simulink model "modelo"  (Simulink 9.1)
settings: Solver=ode15s  StartTime=0.0  StopTime=inf  RelTol=1e-6  EnableMultiTasking=on
libraries: dsparch4 x12, dspmathops x11, dspobslib x7, dspvision x2, dspindex x1
settings Model: Creator=USUARIO  LastModifiedBy=valen
settings DataIOCC: LimitDataPoints=on  SignalLoggingSaveFormat=ModelDataLogs  SignalLoggingName=sigsOut
settings OptimizationCC: ExpressionDepthLimit=2147483647  InitFltsAndDblsToZero=on
settings DebuggingCC: SaveWithParameterizedLinksMsg=none  SignalResolutionControl=TryResolveAllWithWarning  MultiTaskDSMMsg=warning  MultiTaskCondExecSysMsg=none  FcnCallInpInsideContextMsg=warning  StateNameClashWarn=warning
settings HardwareCC: TargetUnknown=on
settings GRTTargetCC: TargetFcnLib=ansi_tfl_tmw.mat

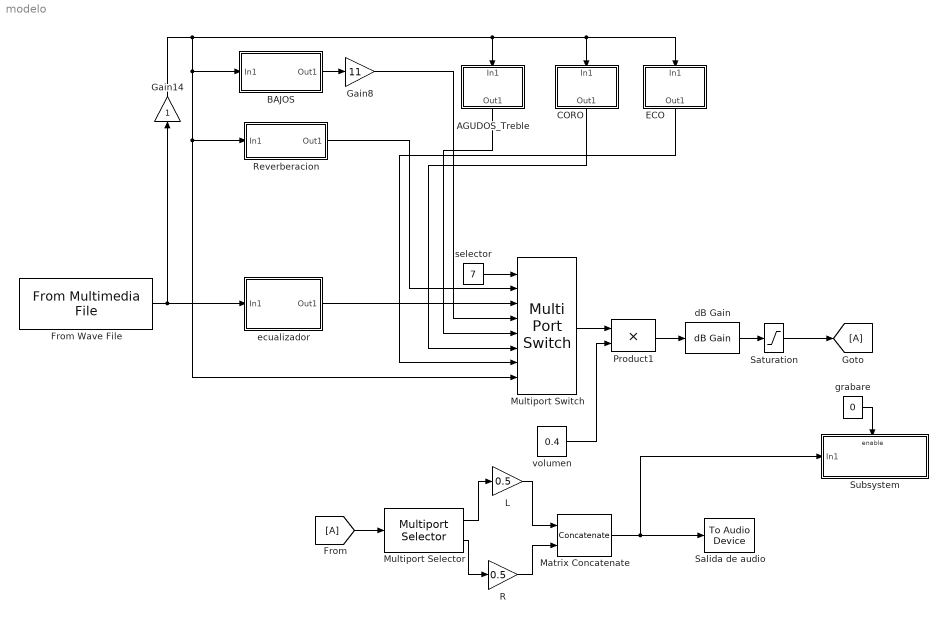
== system modelo ==
  AGUDOS_Treble : Subsystem
  BAJOS : Subsystem
  CORO : Subsystem
  ECO : Subsystem
  From Wave File : dspvision/From Multimedia File  inputFilename=X:\prueba\UNR Ing electrónica\Materias\5.Sistemas y señales I\Unidades\Creo que amo matlab\Ecualizador\5.Ecualizador\LGANTE.wav  loop=on  numPlays=1  outputStreams=Audio only  videoDataType=single  audioDataType=double  inheritSampleTime=on  userDefinedSampleTime=1/30  noAudioOutput=off  isIntensityVideo=off  fourcc=RGB  colorVideoFormat=Separate color signals  outputEOF=off  dataOrg=Column-major  audioFrameSize=256  computeAudioFrameSize=off  outSamplingMode=Frame based
      settings: SourceProductBaseCode=VP
  Gain14 : Gain  SaturateOnIntegerOverflow=on  OutDataTypeStr=Inherit: Same as input  ParamDataTypeStr=Inherit: Same as input
  Gain8 : Gain  Gain=11  SaturateOnIntegerOverflow=on  OutDataTypeStr=Inherit: Same as input  ParamDataTypeStr=Inherit: Same as input
  L : Gain  Gain=0.5
  Matrix Concatenate : Concatenate  Mode=Multidimensional array  ConcatenateDimension=2
  Multiport Selector : dspindex/Multiport Selector  rowsOrCols=Columns  idxCellArray={1,2}  idxErrMode=Clip and Warn
  Multiport Switch : MultiPortSwitch  Inputs=7  SaturateOnIntegerOverflow=on
  Product1 : Product  SaturateOnIntegerOverflow=on  OutDataTypeStr=Inherit: Same as first input
  R : Gain  Gain=0.5
  Reverberacion : Subsystem
  Salida de audio : dspobslib/To Audio Device  deviceName=Default  inheritSampleRate=on  sampleRate=44100  deviceDatatype=Determine from input data type  autoBufferSize=on  bufferSize=4096  queueDuration=2  defaultOutputChannelMapping=on  outputChannelMapping=1:2  outputNumUnderrunSamples=off
      settings: SourceProductName=DSP System Toolbox  SourceProductBaseCode=DS
  Saturation : Saturate  UpperLimit=5  LowerLimit=-5  LinearizeAsGain=off  ZeroCross=off
  Subsystem : Subsystem
  dB Gain : dspmathops/dB Gain  dB=5  intype=Amplitude
      settings: SourceProductName=DSP System Toolbox  SourceProductBaseCode=DS
  ecualizador : Subsystem
  grabare : Constant  Value=0
  selector : Constant  Value=7
  volumen : Constant  Value=0.4
  wires:
  selector/1 -> Multiport Switch/1
  Multiport Switch/1 -> Product1/1
  Product1/1 -> dB Gain/1
  volumen/1 -> Product1/2
  dB Gain/1 -> Saturation/1
  Saturation/1 -> [A]
  From Wave File/1 -> Gain14/1, ecualizador/1(In1)
  Gain14/1 -> AGUDOS_Treble/1(In1), CORO/1(In1), ECO/1(In1), Reverberacion/1(In1), Multiport Switch/8, BAJOS/1(In1)
  Reverberacion/1(Out1) -> Multiport Switch/2
  ecualizador/1(Out1) -> Multiport Switch/3
  BAJOS/1(Out1) -> Gain8/1
  Gain8/1 -> Multiport Switch/4
  AGUDOS_Treble/1(Out1) -> Multiport Switch/5
  CORO/1(Out1) -> Multiport Switch/6
  ECO/1(Out1) -> Multiport Switch/7
  grabare/1 -> Subsystem/Enable
  Multiport Selector/2 -> R/1
  Multiport Selector/1 -> L/1
  L/1 -> Matrix Concatenate/1
  R/1 -> Matrix Concatenate/2
  Matrix Concatenate/1 -> Salida de audio/1, Subsystem/1(In1)
  [A] -> Multiport Selector/1

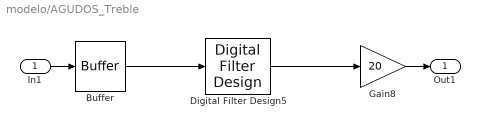
== system modelo/AGUDOS_Treble ==
  In1 : Inport
  Buffer : Buffer  N=256  ic=100
  Digital Filter Design5 : dsparch4/Digital Filter Design  mwdsp_browser_bugfix_var=off
  Gain8 : Gain  Gain=20  SaturateOnIntegerOverflow=on  OutDataTypeStr=Inherit: Same as input  ParamDataTypeStr=Inherit: Same as input
  Out1 : Outport
  wires:
  Buffer/1 -> Digital Filter Design5/1
  Digital Filter Design5/1 -> Gain8/1
  In1/1 -> Buffer/1
  Gain8/1 -> Out1/1

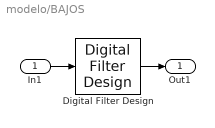
== system modelo/BAJOS ==
  In1 : Inport
  Digital Filter Design : dsparch4/Digital Filter Design  mwdsp_browser_bugfix_var=off
  Out1 : Outport
  wires:
  In1/1 -> Digital Filter Design/1
  Digital Filter Design/1 -> Out1/1

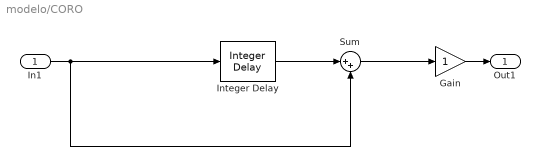
== system modelo/CORO ==
  In1 : Inport
  Gain : Gain  SaturateOnIntegerOverflow=on  OutDataTypeStr=Inherit: Same as input  ParamDataTypeStr=Inherit: Same as input
  Integer Delay : dspobslib/Integer Delay  delay=30e-3*44100  ic=0  reset_popup=None
      settings: SourceProductName=DSP System Toolbox  SourceProductBaseCode=DS
  Sum : Sum  Inputs=|++  SaturateOnIntegerOverflow=on
  Out1 : Outport
  wires:
  In1/1 -> Sum/2, Integer Delay/1
  Integer Delay/1 -> Sum/1
  Sum/1 -> Gain/1
  Gain/1 -> Out1/1

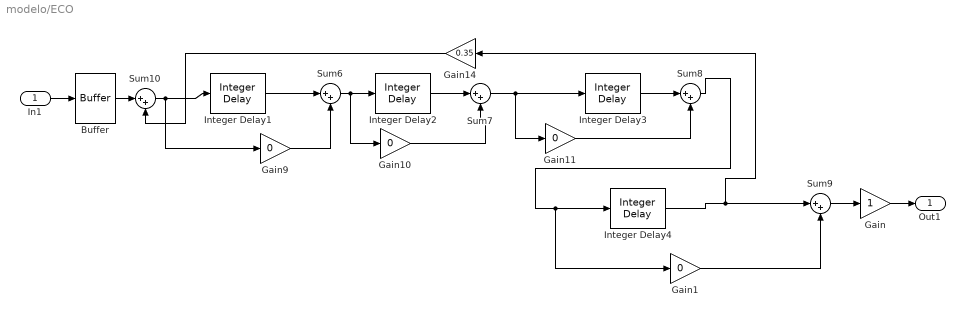
== system modelo/ECO ==
  In1 : Inport
  Buffer : Buffer  N=256  ic=100
  Gain : Gain  SaturateOnIntegerOverflow=on  OutDataTypeStr=Inherit: Same as input  ParamDataTypeStr=Inherit: Same as input
  Gain{1,9..11} (4 alike) : Gain  Gain=0  SaturateOnIntegerOverflow=on  OutDataTypeStr=Inherit: Same as input  ParamDataTypeStr=Inherit: Same as input
  Gain14 : Gain  Gain=0.35  SaturateOnIntegerOverflow=on  OutDataTypeStr=Inherit: Same as input  ParamDataTypeStr=Inherit: Same as input
  Integer Delay{1..4} (4 alike) : dspobslib/Integer Delay  delay=1800  ic=0  reset_popup=None
      settings: SourceProductName=DSP System Toolbox  SourceProductBaseCode=DS
  Sum{6..10} (5 alike) : Sum  Inputs=|++  SaturateOnIntegerOverflow=on
  Out1 : Outport
  wires:
  Integer Delay1/1 -> Sum6/1
  Sum6/1 -> Integer Delay2/1, Gain10/1
  Integer Delay2/1 -> Sum7/1
  Sum7/1 -> Integer Delay3/1, Gain11/1
  Integer Delay3/1 -> Sum8/1
  Gain9/1 -> Sum6/2
  Gain10/1 -> Sum7/2
  Gain11/1 -> Sum8/2
  Sum8/1 -> Integer Delay4/1, Gain1/1
  Integer Delay4/1 -> Sum9/1, Gain14/1
  Sum10/1 -> Integer Delay1/1, Gain9/1
  Gain14/1 -> Sum10/2
  Buffer/1 -> Sum10/1
  Gain1/1 -> Sum9/2
  Sum9/1 -> Gain/1
  In1/1 -> Buffer/1
  Gain/1 -> Out1/1

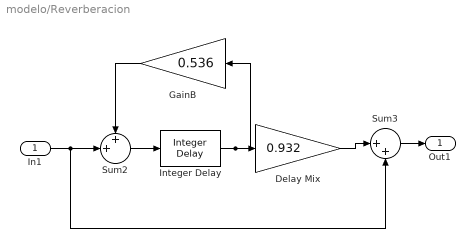
== system modelo/Reverberacion ==
  In1 : Inport
  Delay Mix : Gain  Gain=0.932  SaturateOnIntegerOverflow=on  OutDataTypeStr=Inherit: Same as input  ParamDataTypeStr=Inherit: Same as input
  GainB : Gain  Gain=0.536  SaturateOnIntegerOverflow=on  OutDataTypeStr=Inherit: Same as input  ParamDataTypeStr=Inherit: Same as input
  Integer Delay : dspobslib/Integer Delay  delay=1800  ic=0  reset_popup=None
      settings: SourceProductName=DSP System Toolbox  SourceProductBaseCode=DS
  Sum2 : Sum  Inputs=++|  SaturateOnIntegerOverflow=on  InputSameDT=on  OutDataTypeStr=Inherit: Same as first input
  Sum3 : Sum  Inputs=|++  SaturateOnIntegerOverflow=on  InputSameDT=on  OutDataTypeStr=Inherit: Same as first input
  Out1 : Outport
  wires:
  Sum3/1 -> Out1/1
  In1/1 -> Sum2/2, Sum3/2
  Delay Mix/1 -> Sum3/1
  Integer Delay/1 -> GainB/1, Delay Mix/1
  GainB/1 -> Sum2/1
  Sum2/1 -> Integer Delay/1

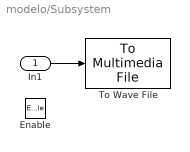
== system modelo/Subsystem ==
  In1 : Inport
  Enable : EnablePort
  To Wave File : dspvision/To Multimedia File  outputFilename=audio_salida.wav  streamSelection=Audio only  videoCompressor=None (uncompressed)  audioCompressor=None (uncompressed)  imagePorts=Separate color signals  fileType=WAV  audioDatatype=16-bit integer  fourcc=RGB  videoQuality=75  mj2000CompFactor=10
      settings: SourceProductName=DSP System Toolbox  SourceProductBaseCode=DS
  wires:
  In1/1 -> To Wave File/1

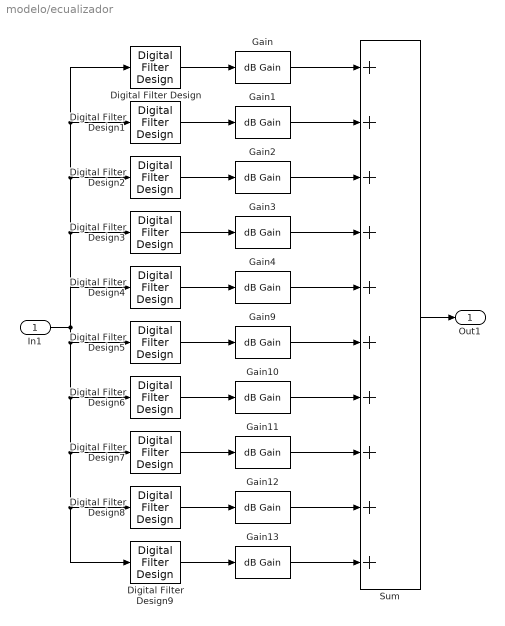
== system modelo/ecualizador ==
  In1 : Inport
  Digital Filter Design{,1..9} (10 alike) : dsparch4/Digital Filter Design  mwdsp_browser_bugfix_var=off
  Gain : dspmathops/dB Gain  dB=4  intype=Amplitude
      settings: SourceProductName=DSP System Toolbox  SourceProductBaseCode=DS
  Gain1 : dspmathops/dB Gain  dB=3  intype=Amplitude
      settings: SourceProductName=DSP System Toolbox  SourceProductBaseCode=DS
  Gain10 : dspmathops/dB Gain  dB=4  intype=Amplitude
      settings: SourceProductName=DSP System Toolbox  SourceProductBaseCode=DS
  Gain11 : dspmathops/dB Gain  dB=5  intype=Amplitude
      settings: SourceProductName=DSP System Toolbox  SourceProductBaseCode=DS
  Gain12 : dspmathops/dB Gain  dB=5  intype=Amplitude
      settings: SourceProductName=DSP System Toolbox  SourceProductBaseCode=DS
  Gain13 : dspmathops/dB Gain  dB=5  intype=Amplitude
      settings: SourceProductName=DSP System Toolbox  SourceProductBaseCode=DS
  Gain2 : dspmathops/dB Gain  dB=0  intype=Amplitude
      settings: SourceProductName=DSP System Toolbox  SourceProductBaseCode=DS
  Gain3 : dspmathops/dB Gain  dB=-2  intype=Amplitude
      settings: SourceProductName=DSP System Toolbox  SourceProductBaseCode=DS
  Gain4 : dspmathops/dB Gain  dB=-2  intype=Amplitude
      settings: SourceProductName=DSP System Toolbox  SourceProductBaseCode=DS
  Gain9 : dspmathops/dB Gain  dB=0  intype=Amplitude
      settings: SourceProductName=DSP System Toolbox  SourceProductBaseCode=DS
  Sum : Sum  Inputs=++++++++++  SaturateOnIntegerOverflow=on
  Out1 : Outport
  wires:
  In1/1 -> Digital Filter Design4/1, Digital Filter Design/1, Digital Filter Design1/1, Digital Filter Design2/1, Digital Filter Design3/1, Digital Filter Design5/1, Digital Filter Design6/1, Digital Filter Design7/1, Digital Filter Design9/1, Digital Filter Design8/1
  Sum/1 -> Out1/1
  Digital Filter Design/1 -> Gain/1
  Digital Filter Design1/1 -> Gain1/1
  Digital Filter Design2/1 -> Gain2/1
  Digital Filter Design3/1 -> Gain3/1
  Digital Filter Design4/1 -> Gain4/1
  Digital Filter Design5/1 -> Gain9/1
  Digital Filter Design6/1 -> Gain10/1
  Digital Filter Design7/1 -> Gain11/1
  Digital Filter Design8/1 -> Gain12/1
  Digital Filter Design9/1 -> Gain13/1
  Gain/1 -> Sum/1
  Gain1/1 -> Sum/2
  Gain2/1 -> Sum/3
  Gain3/1 -> Sum/4
  Gain4/1 -> Sum/5
  Gain9/1 -> Sum/6
  Gain10/1 -> Sum/7
  Gain11/1 -> Sum/8
  Gain12/1 -> Sum/9
  Gain13/1 -> Sum/10
